simulink model "speed"  (R2024b)
settings: Solver=VariableStepAuto  StartTime=0.0  StopTime=10.0  RelTol=1e-3
undefined symbols (not defined in the file): Clink, DiscIntNeverNeededParam, phi_n, RBrake, Switch_off_point, Switch_on_point, Ts_Power
libraries: spsStairGeneratorLib x3, spsSeriesRLCBranchLib x2, spsThreePhaseVIMeasurementLib x2, spsAsynchronousMachinepuUnitsLib x1, spsIGBTLib x1, spsVoltageMeasurementLib x1, simulink x1, dspsigops x1, eeGeneralControl x1, eeAsmDtcSvm x1, spsThreePhaseSourceLib x1, spsTwoLevelConverterLib x1
settings Model: Creator=asus  LastModifiedBy=asus

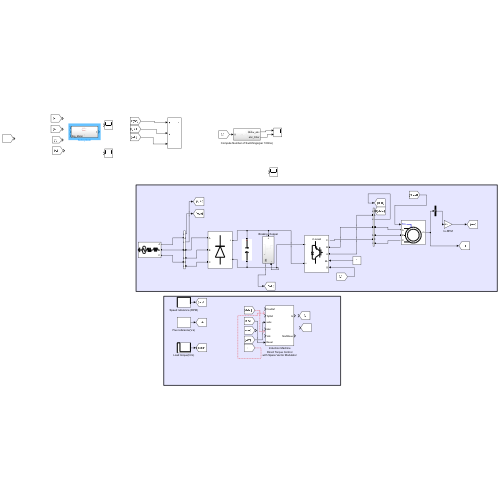
[thumbnail: Simulink's stored preview of the top-level diagram]
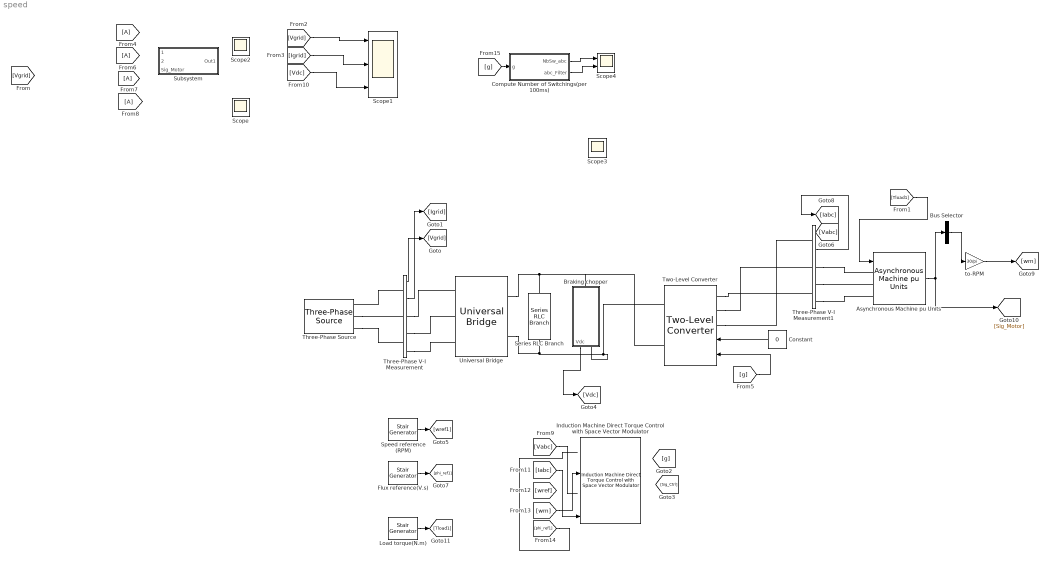
== system speed ==
  Asynchronous Machine pu Units : spsAsynchronousMachinepuUnitsLib/Asynchronous Machine pu Units  RotorType=Squirrel-cage  PresetModel=No  MechanicalLoad=Torque Tm  ShowDetailedParameters=on  ReferenceFrame=Rotor  Units=pu  MeasurementBus=off  NominalParameters=[3730 460 60]  VoltageRatio=1  Stator=[0.01965 0.0397]  Rotor=[0.01909 0.0397]  Cage1=[0.01909 0.0397]  Cage2=[0.01909 0.0397]  Lm=1.354  Mechanical=[0.09526 0.05479 2]  PolePairs=2  InitialConditions="[ 1,0   0,0,0   0,0,0 ]"  SimulateSaturation=off  Saturation="[0.212,0.4201,0.8125,1.0979,1.4799,2.2457,3.2586,4.5763,6.4763 ;   0.5,0.7,0.9,1,1.1,1.2 ,1.3,1.4,1.5]"  LoadFlowParameters=0  TsPowergui=0  TsBlock=-1  IterativeModel=Trapezoidal non iterative  IterativeDiscreteModel=Trapezoidal non iterative  Pmec=0
      settings: LibrarySourceBlock=|
      | sps_lib/Electrical Machines/Asynchronous Machine
      | pu Units
  Braking chopper : Subsystem
      settings: PortSchema="{\"entries\":[{\"content\":{\"sides\":[{\"content\":{\"connectorIds\":[\"Out1\",\"LConn1\"]},\"type\":\"ConnectorPlacement.EquallySpacedRectSide\",\"uuid\":\"c6780781-d710-476a-a877-7eecf153e931\"},{\"content\":{\"connectorIds\":[\"RConn1\"],\"side\":\"RIGHT\"},\"type\":\"ConnectorPlacement.EquallySpacedRectSide\",\"uuid\":\"cc9bff95-ede1-4626-a915-44a14f61ad98\"},{\"content\":{\"side\":\"TOP\"},\"type\":\"ConnectorPlacement.EquallySpacedRectSide\",\"uuid\":\"a71c811e-9ed7-4d07-a57c-1628f4980a10\"},{\"content\":{\"side\":\"BOTTOM\"},\"type\":\"ConnectorPlacement.EquallySpacedRectSide\",\"uuid\":\"3f3fd56f-6316-494b-bf18-08be0d9b555f\"}]},\"type\":\"ConnectorPlacement.EquallySpacedConnector\",\"uuid\":\"9b82ef15-cf2b-465d-8942-3536d499c5d1\"}],\"packageUris\":[\"http://schema.mathworks.com/mf0/Connector/R2020b\"],\"version\":\"1.0\"}"
  Bus Selector : BusSelector  OutputSignals=Mechanical.Rotor speed (wm)  OutputAsBus=on
  Compute Number of Switchings(per 100ms) : Subsystem
  Constant : Constant  Value=0  SampleTime=Ts_Power
  Flux reference(V.s) : spsStairGeneratorLib/Stair Generator  t=[0 3.5]  e=[phi_n*0.9 phi_n*1.0]  Ts=Ts_Power
  From{4,6..8} (4 alike) : From
  Induction Machine Direct Torque Control with Space Vector Modulator : eeAsmDtcSvm/Induction Machine Direct Torque Control with Space Vector Modulator  Rs=0.25  p=1  Vdc_on=300  Ts=5e-6  Tsc=5e-5  fsw=1000  Kp_flux=150  Ki_flux=3000  Kaw_flux=1  Kp_tq=1  Ki_tq=50  Kaw_tq=1  AxisPrio=Q-axis
      settings: LibrarySourceBlock=|
      | ee_sl_lib/Induction Machine
      | Control/Induction Machine
      | Direct Torque Control
      | with Space Vector Modulator
  Load torque(N.m) : spsStairGeneratorLib/Stair Generator  t=[0 1.5 2.0 4]  e="[0 500 50  500]"  Ts=Ts_Power
  Scope : Scope
  Scope1 : Scope  NumInputPorts=3
  Scope2 : Scope
  Scope3 : Scope
  Scope4 : Scope  NumInputPorts=2
  Series RLC Branch : spsSeriesRLCBranchLib/Series RLC Branch  LConnTagsString=__new0  RConnTagsString=__new0  BranchType=C  Resistance=1  Inductance=1e-3  SetiL0=off  InitialCurrent=0  Capacitance=Clink  Setx0=on  InitialVoltage=640  Measurements=None
  Speed reference (RPM) : spsStairGeneratorLib/Stair Generator  t="[0  0.1  2.5]"  e=[0 1500 500]  Ts=Ts_Power
  Subsystem : Subsystem
  Three-Phase V-I Measurement : spsThreePhaseVIMeasurementLib/Three-Phase V-I Measurement  VoltageMeasurement=phase-to-ground  SetLabelV=off  LabelV=Vabc  Vpu=off  VpuLL=off  CurrentMeasurement=yes  SetLabelI=off  LabelI=Iabc  Ipu=off  Pbase=100e6  Vbase=500e3  OutputType=Complex  PhasorSimulation=off  PSBequivalent=0
  Three-Phase V-I Measurement1 : spsThreePhaseVIMeasurementLib/Three-Phase V-I Measurement  VoltageMeasurement=phase-to-ground  SetLabelV=off  LabelV=Vabc  Vpu=off  VpuLL=off  CurrentMeasurement=yes  SetLabelI=off  LabelI=Iabc  Ipu=off  Pbase=100e6  Vbase=500e3  OutputType=Complex  PhasorSimulation=off  PSBequivalent=0
  Three-Phase Source : spsThreePhaseSourceLib/Three-Phase Source  InternalConnection=Yg  VoltagePhases=off  Voltage=460  PhaseAngle=0  Voltage_phases=[25e3 25e3 25e3]/sqrt(3)  PhaseAngles_phases=[0 -120 +120]  Frequency=60  NonIdealSource=on  SpecifyImpedance=off  Resistance=0.01  Inductance=0.025e-3  ShortCircuitLevel=100e6  BaseVoltage=460  XRratio=7  BusType=swing  Pref=10e3  Qref=0  Prefabc=[10e3, 10e3, 10e3]  Qrefabc=[0, 0, 0]  Qmin=-inf  Qmax=inf
  Two-Level Converter : spsTwoLevelConverterLib/Two-Level Converter  ModelType=Switching devices  Ron=1e-3  Rs=1e6  Cs=inf  Vforward=[0,0]  Ron_Diode=1e-3  Rs_Diode=1e6  Cs_Diode=inf  Vf_Diode=1e-3  Rs_CurrentSource=inf  Ron_ACsource=1e-3
      settings: LibrarySourceBlock=sps_lib/Power Electronics/Two-Level Converter
  Universal Bridge : spsUniversalBridgeLib/Universal Bridge  Arms=3  SnubberResistance=1e6  SnubberCapacitance=inf  Device=Diodes  Ron=1e-3  Lon=0  ForwardVoltages="[  0  0  ]"  ForwardVoltage=0  GTOparameters=[ 10e-6 , 20e-6 ]  IGBTparameters=[ 1e-6 , 2e-6 ]  Measurements=None  Measurements_2=None  converterType=Rectifier
  to-RPM : Gain  Gain=30/pi
  wires:
  Three-Phase V-I Measurement/1 -> [Vgrid]
  Three-Phase V-I Measurement/2 -> [Igrid]
  Braking chopper/1(Vdc) -> [Vdc]
  [g] -> Two-Level Converter/1
  Constant/1 -> Two-Level Converter/2
  Three-Phase V-I Measurement1/1 -> [Vabc]
  Three-Phase V-I Measurement1/2 -> [Iabc]
  [Tload1] -> Asynchronous Machine pu Units/1
  to-RPM/1 -> [wm]
  Asynchronous Machine pu Units/1 -> [Sig_Motor], Bus Selector/1
  Bus Selector/1 -> to-RPM/1
  [Vgrid] -> Scope1/1
  [Vdc] -> Scope1/3
  [Igrid] -> Scope1/2
  [g] -> Compute Number of Switchings(per 100ms)/1(g)
  Compute Number of Switchings(per 100ms)/1(NbSw_abc) -> Scope4/1
  Compute Number of Switchings(per 100ms)/2(abc_Filter) -> Scope4/2
  Speed reference (RPM)/1 -> [wref1]
  Flux reference(V.s)/1 -> [phi_ref1]
  Load torque(N.m)/1 -> [Tload1]
  [Vabc] -> ?
  [Iabc] -> Induction Machine Direct Torque Control with Space Vector Modulator/6
  [wm] -> Induction Machine Direct Torque Control with Space Vector Modulator/3
  [phi_ref1] -> ?
  connections:
  Three-Phase V-I Measurement/LConn1 -- Three-Phase Source/RConn1
  Three-Phase Source/RConn2 -- Three-Phase V-I Measurement/LConn2
  Three-Phase Source/RConn3 -- Three-Phase V-I Measurement/LConn3
  Three-Phase V-I Measurement/RConn3 -- Universal Bridge/LConn3
  Three-Phase V-I Measurement/RConn2 -- Universal Bridge/LConn2
  Three-Phase V-I Measurement/RConn1 -- Universal Bridge/LConn1
  Universal Bridge/RConn1 -- Two-Level Converter/RConn1 -- Braking chopper/RConn1 -- Series RLC Branch/LConn1
  Universal Bridge/RConn2 -- Two-Level Converter/RConn2 -- Braking chopper/LConn1 -- Series RLC Branch/RConn1
  Two-Level Converter/LConn1 -- Three-Phase V-I Measurement1/LConn1
  Two-Level Converter/LConn2 -- Three-Phase V-I Measurement1/LConn2
  Two-Level Converter/LConn3 -- Three-Phase V-I Measurement1/LConn3
  Three-Phase V-I Measurement1/RConn1 -- Asynchronous Machine pu Units/LConn1
  Three-Phase V-I Measurement1/RConn2 -- Asynchronous Machine pu Units/LConn2
  Three-Phase V-I Measurement1/RConn3 -- Asynchronous Machine pu Units/LConn3

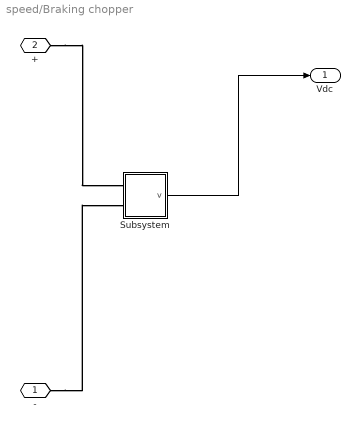
== system speed/Braking chopper ==
  Subsystem : Subsystem
  - : PMIOPort  Side=Left
  + : PMIOPort  Port=2  Side=Right
  Vdc : Outport
  wires:
  Subsystem/1(v) -> Vdc/1
  connections:
  +/RConn1 -- Subsystem/LConn1
  -/RConn1 -- Subsystem/LConn2

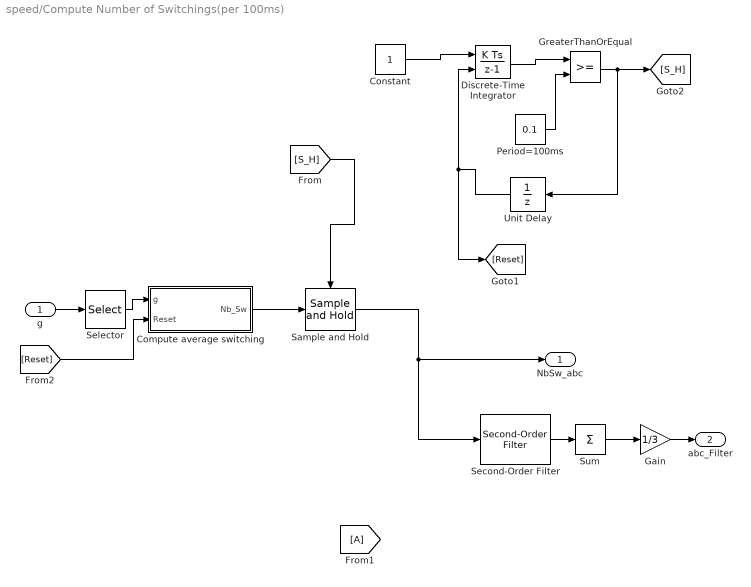
== system speed/Compute Number of Switchings(per 100ms) ==
  g : Inport
  Compute average switching : Subsystem
  Constant : Constant
  Discrete-Time Integrator : DiscreteIntegrator  ExternalReset=rising  SampleTime=Ts_Power  ICPrevOutput=DiscIntNeverNeededParam  ICPrevScaledInput=DiscIntNeverNeededParam
  From1 : From
  Gain : Gain  Gain=1/3
  GreaterThanOrEqual : RelationalOperator  OutDataTypeStr=boolean  RndMeth=Simplest  InputSameDT=off
  Period=100ms : Constant  Value=0.1
  Sample and Hold : dspsigops/Sample and Hold  trig=Rising edge  initCond=0  latchinput=off
  Second-Order Filter : eeGeneralControl/Second-Order Filter  FilterType=Low-pass  fn=5  Zeta=1  Ts=Ts_Power  A0=0  Ph0=0  f0=0  b0=0
      settings: LibrarySourceBlock=ee_sl_lib/General Control/Second-Order Filter
  Selector : Selector  InputPortWidth=6  IndexOptions=Index vector (dialog)  Indices=[1 3 5]  OutputSizes=1
  Sum : Sum  Inputs=+
  Unit Delay : UnitDelay  SampleTime=-1  HasFrameUpgradeWarning=on
  NbSw_abc : Outport
  abc_Filter : Outport  Port=2
  wires:
  g/1 -> Selector/1
  Constant/1 -> Discrete-Time Integrator/1
  GreaterThanOrEqual/1 -> Unit Delay/1, [S_H]
  Discrete-Time Integrator/1 -> GreaterThanOrEqual/1
  Period=100ms/1 -> GreaterThanOrEqual/2
  Unit Delay/1 -> Discrete-Time Integrator/2, [Reset]
  [S_H] -> Sample and Hold/Trigger
  Sample and Hold/1 -> Second-Order Filter/1, NbSw_abc/1
  Second-Order Filter/1 -> Sum/1
  Sum/1 -> Gain/1
  Gain/1 -> abc_Filter/1
  Selector/1 -> Compute average switching/1(g)
  Compute average switching/1(Nb_Sw) -> Sample and Hold/1
  [Reset] -> Compute average switching/2(Reset)

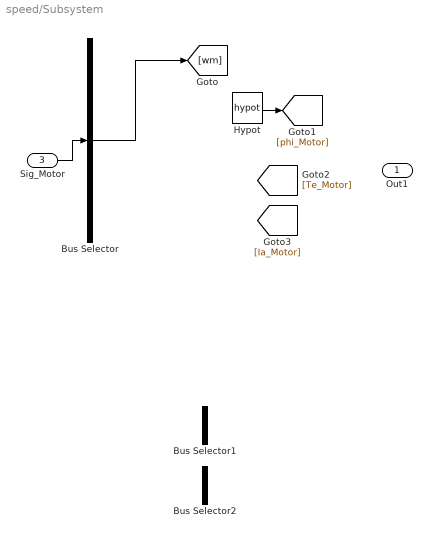
== system speed/Subsystem ==
  Sig_Motor : Inport  Port=3
  Bus Selector : BusSelector  OutputSignals=mechanical,stator flux phis_q,signal1,electromagnetic torque Te(N*m),signal2  OutputAsBus=on
  Bus Selector1 : BusSelector  OutputSignals=signal1,signal2
  Bus Selector2 : BusSelector  OutputSignals=Mechanical.Rotor speed (wm)  OutputAsBus=on
  Hypot : Math  Operator=hypot
  Out1 : Outport
  wires:
  Sig_Motor/1 -> Bus Selector/1
  Bus Selector/1 -> [wm]
  Hypot/1 -> [phi_Motor]
  ? -> Hypot/2  "<signal1>"
  ? -> [Ia_Motor]  "<signal2>"
  ? -> Hypot/1  "<stator flux phis_q>"
  ? -> [Te_Motor]  "<electromagnetic torque Te(N*m)>"

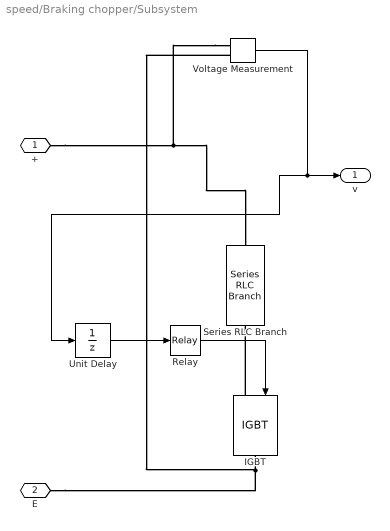
== system speed/Braking chopper/Subsystem ==
  IGBT : spsIGBTLib/IGBT  Ron=1e-3  Lon=0  Vf=0  Tf=1e-6  Tt=2e-6  IC=0  Rs=1e6  Cs=inf  Measurements=off
  Relay : Relay  OnSwitchValue=Switch_on_point  OffSwitchValue=Switch_off_point  OutDataTypeStr=double
  Series RLC Branch : spsSeriesRLCBranchLib/Series RLC Branch  LConnTagsString=__new0  RConnTagsString=__new0  BranchType=R  Resistance=RBrake  Inductance=1e-3  SetiL0=off  InitialCurrent=0  Capacitance=1e-6  Setx0=off  InitialVoltage=0  Measurements=None
  Unit Delay : UnitDelay  SampleTime=-1  HasFrameUpgradeWarning=on
  Voltage Measurement : spsVoltageMeasurementLib/Voltage Measurement  PhasorSimulation=off  OutputType=Complex  PSBequivalent=0
  + : PMIOPort  Side=Left
  E : PMIOPort  Port=2  Side=Left
  v : Outport
  wires:
  Unit Delay/1 -> Relay/1
  Voltage Measurement/1 -> v/1, Unit Delay/1
  Relay/1 -> IGBT/1
  connections:
  Voltage Measurement/LConn1 -- Series RLC Branch/LConn1 -- +/RConn1
  IGBT/RConn1 -- E/RConn1 -- Voltage Measurement/LConn2
  IGBT/LConn1 -- Series RLC Branch/RConn1

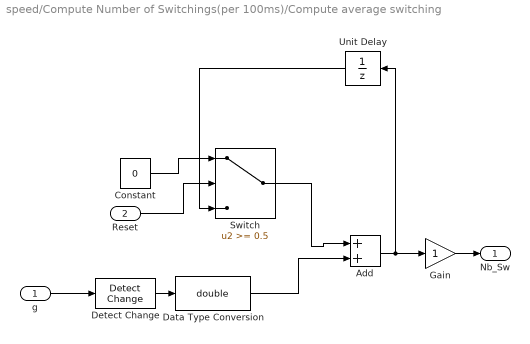
== system speed/Compute Number of Switchings(per 100ms)/Compute average switching ==
  g : Inport
  Reset : Inport  Port=2
  Add : Sum
  Constant : Constant  Value=0
  Data Type Conversion : DataTypeConversion  OutDataTypeStr=double  SaturateOnIntegerOverflow=off  RndMeth=Floor
  Detect Change : simulink/Logic and Bit Operations/Detect Change  vinit=0  OutDataTypeStr=boolean
  Gain : Gain
  Switch : Switch  Threshold=0.5  SaturateOnIntegerOverflow=off  InputSameDT=off
  Unit Delay : UnitDelay  SampleTime=-1  HasFrameUpgradeWarning=on
  Nb_Sw : Outport
  wires:
  g/1 -> Detect Change/1
  Constant/1 -> Switch/1
  Reset/1 -> Switch/2
  Unit Delay/1 -> Switch/3
  Switch/1 -> Add/1
  Add/1 -> Unit Delay/1, Gain/1
  Detect Change/1 -> Data Type Conversion/1
  Gain/1 -> Nb_Sw/1
  Data Type Conversion/1 -> Add/2
